simulink model "chap7_3"  (Simulink 3.00)
settings: Solver=ode45  StartTime=0.0  StopTime=100  RelTol=1e-3
values from neighbouring files (symbols this model uses):
  a1 = 20    [chap7_16.m]    (also in chap7_16eq.m = para(1); chap7_3f.m = 3)
  a2 = 43    [chap7_3f.m]
  kd = 0.20    (= 0.2)    [chap7_10.m]    (also in chap7_14.m = 0.01; chap7_15f.m = 1; chap7_2.m = 15; chap7_3f.m = 1.9688)
  ki = 0.80    (= 0.8)    [chap7_10.m]    (also in chap7_14.m = 0.01; chap7_15f.m = 10; chap7_2.m = 0; chap7_3f.m = 0.0504)
  kp = 8.0    (= 8)    [chap7_10.m]    (also in chap7_14.m = 0.1; chap7_15f.m = 50; chap7_2.m = 50; chap7_3f.m = 0.63)
libraries: simulink_extras x1

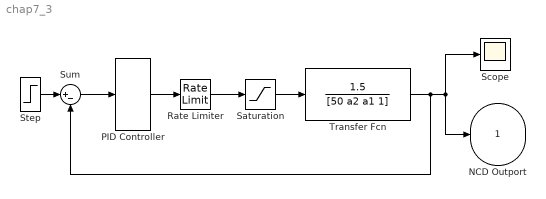
== system chap7_3 ==
  PID Controller : simulink_extras/Additional Linear/PID Controller  P=kp  I=ki  D=kd
  Rate Limiter : RateLimiter  RisingSlewLimit=0.8  FallingSlewLimit=-0.8
  Saturation : Saturate  UpperLimit=1  LowerLimit=-1
  Scope : Scope
      settings: TimeRange=auto  YMin=-5  YMax=5  SaveToWorkspace=off  SaveName=ScopeData
  Step : Step  Time=1  Before=0  After=1  SampleTime=0
  Sum : Sum  Inputs=|+-  SaturateOnIntegerOverflow=on
  Transfer Fcn : TransferFcn  Numerator=[1.5]  Denominator=[50 a2 a1 1]
  NCD Outport : Outport  Port=1  InitialOutput=0
      settings: OpenFcn=optblock
      mask Type: NCD Outport
      mask Display:
      | plot([0:10],[-.5 1.5 .6 1.3 .8 1.1 .95 1.02 .99 1 1]);
      | disp('\n\n NCD\n OutPort 1');
  wires:
  Sum/1 -> PID Controller/1
  Step/1 -> Sum/1
  PID Controller/1 -> Rate Limiter/1
  Rate Limiter/1 -> Saturation/1
  Saturation/1 -> Transfer Fcn/1
  Transfer Fcn/1 -> NCD Outport/1, Scope/1, Sum/2
